simulink subsystem "Track_Drag_Coefficents"  (R2023a)
settings: Solver=VariableStepAuto  StartTime=0.0  StopTime=10.0  RelTol=1e-3
undefined symbols (not defined in the file): covariance, twist
libraries: ros2lib x2

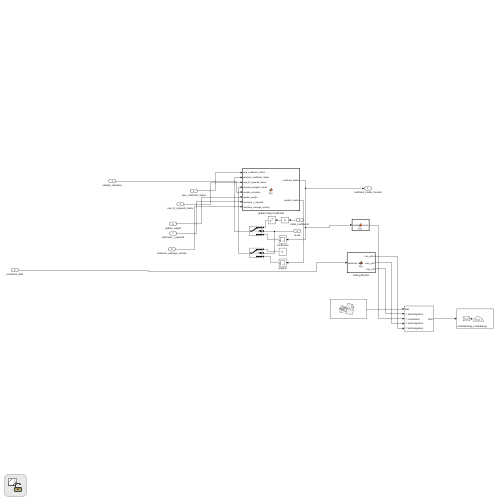
[thumbnail: Simulink's stored preview of the top-level diagram]
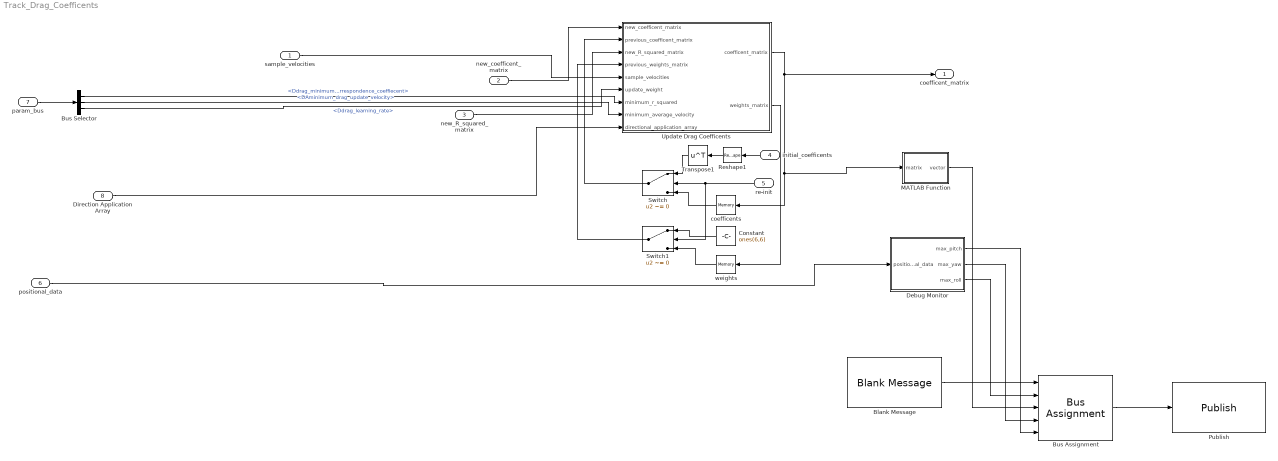
== system Track_Drag_Coefficents ==
  sample_velocities : Inport
  new_coefficent_matrix : Inport  Port=2
  new_R_squared_matrix : Inport  Port=3
  initial_coefficents : Inport  Port=4
  re-init : Inport  Port=5
  positional_data : Inport  Port=6
  param_bus : Inport  Port=7
  Direction Application Array : Inport  Port=8
  Blank Message : ros2lib/Blank Message  messageClass=Message  entityType=geometry_msgs/TwistWithCovariance  messageType=geometry_msgs/TwistWithCovariance  SampleTime=inf
  Bus Assignment : BusAssignment  AssignedSignals=twist.angular.x,covariance,twist.angular.z,twist.angular.y
  Bus Selector : BusSelector  OutputSignals=Ddrag_minimum_correspondence_coeffiecent,DAminimum_drag_update_velocity,Ddrag_learning_rate
  Constant : Constant  Value=ones(6,6)
  Debug Monitor : MATLAB Function  TreatAsAtomicUnit=on
  MATLAB Function : MATLAB Function  TreatAsAtomicUnit=on
  Publish : ros2lib/Publish  topicSource=Specify your own  topic=/controller/drag_comp/debug  messageType=geometry_msgs/TwistWithCovariance  QOSHistory=Keep last  QOSDepth=1  QOSReliability=Reliable  QOSDurability=Volatile
  Reshape1 : Reshape  OutputDimensionality=Customize  OutputDimensions=[6,6]
  Switch : Switch  Criteria=u2 ~= 0  SaturateOnIntegerOverflow=off  InputSameDT=off
  Switch1 : Switch  Criteria=u2 ~= 0  SaturateOnIntegerOverflow=off  InputSameDT=off
  Transpose1 : Math  Operator=transpose
  Update Drag Coefficents : MATLAB Function  TreatAsAtomicUnit=on
  coefficents : Memory  InitialCondition=zeros(6,6)
  weights : Memory  InitialCondition=ones(6,6)
  coefficent_matrix : Outport
  wires:
  Debug Monitor/2(max_yaw) -> Bus Assignment/4
  Bus Assignment/1 -> Publish/1
  positional_data/1 -> Debug Monitor/1(positional_data)
  weights/1 -> Switch1/3
  Constant/1 -> Switch1/1
  new_R_squared_matrix/1 -> Update Drag Coefficents/3(new_R_squared_matrix)
  new_coefficent_matrix/1 -> Update Drag Coefficents/1(new_coefficent_matrix)
  initial_coefficents/1 -> Reshape1/1
  sample_velocities/1 -> Update Drag Coefficents/5(sample_velocities)
  Update Drag Coefficents/2(weights_matrix) -> weights/1
  Update Drag Coefficents/1(coefficent_matrix) -> MATLAB Function/1(matrix), coefficents/1, coefficent_matrix/1
  Switch1/1 -> Update Drag Coefficents/4(previous_weights_matrix)
  MATLAB Function/1(vector) -> Bus Assignment/3
  Switch/1 -> Update Drag Coefficents/2(previous_coefficent_matrix)
  Reshape1/1 -> Transpose1/1
  coefficents/1 -> Switch/3
  Transpose1/1 -> Switch/1
  Debug Monitor/1(max_pitch) -> Bus Assignment/5
  Debug Monitor/3(max_roll) -> Bus Assignment/2
  re-init/1 -> Switch/2, Switch1/2
  Blank Message/1 -> Bus Assignment/1
  param_bus/1 -> Bus Selector/1
  Bus Selector/1 -> Update Drag Coefficents/7(minimum_r_squared)  "<Ddrag_minimum_correspondence_coeffiecent>"
  Bus Selector/2 -> Update Drag Coefficents/8(minimum_average_velocity)  "<DAminimum_drag_update_velocity>"
  Bus Selector/3 -> Update Drag Coefficents/6(update_weight)  "<Ddrag_learning_rate>"
  Direction Application Array/1 -> Update Drag Coefficents/9(directional_application_array)

== matlab function Track_Drag_Coefficents/MATLAB Function ==
function vector = fcn(matrix)

vector = [matrix(1,:),matrix(2,:),matrix(3,:),matrix(4,:),matrix(5,:),matrix(6,:)]';

== matlab function Track_Drag_Coefficents/Update Drag Coefficents ==
function [coefficent_matrix, weights_matrix] = fcn(new_coefficent_matrix, previous_coefficent_matrix, new_R_squared_matrix, previous_weights_matrix, sample_velocities, update_weight, minimum_r_squared, minimum_average_velocity, directional_application_array)

weights_matrix = previous_weights_matrix;
coefficent_matrix = previous_coefficent_matrix;

    for correction_axis = 1:6
        for motion_axis = 1:6
            if(new_R_squared_matrix(correction_axis, motion_axis) > minimum_r_squared && abs(mean(sample_velocities(motion_axis,:))) > minimum_average_velocity(motion_axis) && directional_application_array(motion_axis))
                
                weights_matrix(correction_axis, motion_axis) = previous_weights_matrix(correction_axis, motion_axis) + new_R_squared_matrix(correction_axis, motion_axis) * update_weight;
                
                coefficent_matrix(correction_axis, motion_axis) = (new_coefficent_matrix(correction_axis, motion_axis) * new_R_squared_matrix(correction_axis, motion_axis) * update_weight + previous_coefficent_matrix(correction_axis, motion_axis) * previous_weights_matrix(correction_axis, motion_axis)) / ...
                    weights_matrix(correction_axis, motion_axis);
            end
        end
    end


end

== matlab function Track_Drag_Coefficents/Debug Monitor ==
function [max_pitch, max_yaw, max_roll] = fcn(positional_data)

eul_angles = quat2eul([positional_data(7,:)', positional_data(4,:)',positional_data(5,:)',positional_data(6,:)'], 'XYZ');

max_roll = max(abs(eul_angles(:,3)));
max_pitch = max(abs(eul_angles(:,2)));
max_yaw = max(abs(eul_angles(:,1)));
